simulink model "IOT_Charger"  (R2024b)
settings: Solver=ode23tb  StartTime=0.0  StopTime=1  RelTol=1e-3  EnableMultiTasking=on
PreLoadFcn:
  | % Data of Solar Panel
  | %5000[W]/130[W]
  | % Total power generated by solar panel reaches 5[KW].
  | % each solar panel generates power 130[kW].
  | V = [0    40 80 120 160 180 200 217 240 260 280];
  | I = 5000/130*[0.68 0.675 0.67 0.665 0.660 0.655 0.640 0.6 0.48 0.28 0];
  | 
  | %subplot(211);plot(V,I);xlabel('Voltage[V]');ylabel('Current[a]')
  | %subplot(212);plot(V.*I);title('Power[W]')
  | 
  | % Sample Time[s]
  | Ts =5e-6;
  | 
  | 
  | %MPPT + PV Control
  | % PI control pamameter of Voltage control(Outer loop)
  | Kp_V = 50e-3;
  | Ki_V = 10;
  | 
  | % PI Control pamameter of Current control(Inner loop)
  | Kp_I = 25e-3;
  | Ki_I = 10;
  | 
  | % Utility Interconnection Control
  | % PI Control pamameter of Voltage control(Outer loop)
  | Kp_V2 = 0.01;
  | Ki_V2 = 25;
  | 
  | % PI control pamameter of Current control(Inner loop)
  | Kp_I2 = 0.01;
  | Ki_I2 = 25;
  | 
  | 
  | % Difference of voltege using in MPPT
  | dV = 0.5;
  | 
  | % Battery Control
  | % PI Control pamameter of Voltage control(Outer loop)
  | Kp_VB = 0.4;
  | Ki_VB = 2;
  | 
  | % PI control pamameter of Current control(Inner loop)
  | Kp_IB = 0.1;
  | Ki_IB = 0.5;
undefined symbols (not defined in the file): Ion, Lithium, sigbuilder_block
libraries: spsBreakerLib x120, spsSeriesRLCBranchLib x72, spsBatteryLib x43, spsIdealSwitchLib x29, spsVoltageMeasurementLib x25, spsMosfetLib x19, slpidlib x17, spsSeriesRLCLoadLib x12, spsPWMGeneratorDCDCLib x11, spsCurrentMeasurementLib x10, spsDiodeLib x6, spsPWMGenerator2LevelLib x5
(part 6 of 6)

== matlab function IOT_Charger/MPPT and PV Controller/Swapping battery controller/MATLAB Function17 ==
  settings: updateMethod=DISCRETE
  data: SOC input; LoadOn output; ChargingOn output
function [LoadOn, ChargingOn] = chargeDischargeNode(SOC)
    % This function determines the charging and discharging states
    % based on the state of charge (SOC) of the battery.
    % Inputs:
    %   SOC - Current state of charge (0 to 100)
    % Outputs:
    %   LoadOn - Indicator if the load is on (1) or off (0)
    %   ChargingOn - Indicator if charging is active (1) or not (0)

    % Initialize persistent variables to retain state across function calls
    persistent LoadOnPersistent;
    persistent ChargingOnPersistent;

    if isempty(LoadOnPersistent)  % Initialize on first call
        LoadOnPersistent = 1;     % Load is initially on
        ChargingOnPersistent = 0;  % Charging is initially off
    end

    % Logic for charging and discharging based on SOC levels
    if SOC > 80
        LoadOnPersistent = 1;      % Turn load on if SOC is above 80%
        ChargingOnPersistent = 0;   % Turn charging off
    elseif SOC < 40
        LoadOnPersistent = 0;      % Turn load off if SOC is below 40%
        ChargingOnPersistent = 1;   % Start charging
    end

    % Assign output values from persistent variables
    LoadOn = LoadOnPersistent;
    ChargingOn = ChargingOnPersistent;
end

== matlab function IOT_Charger/MPPT and PV Controller/Swapping battery controller/MATLAB Function18 ==
  settings: updateMethod=DISCRETE
  data: SOC input; LoadOn output; ChargingOn output
function [LoadOn, ChargingOn] = chargeDischargeNode(SOC)
    % This function determines the charging and discharging states
    % based on the state of charge (SOC) of the battery.
    % Inputs:
    %   SOC - Current state of charge (0 to 100)
    % Outputs:
    %   LoadOn - Indicator if the load is on (1) or off (0)
    %   ChargingOn - Indicator if charging is active (1) or not (0)

    % Initialize persistent variables to retain state across function calls
    persistent LoadOnPersistent;
    persistent ChargingOnPersistent;

    if isempty(LoadOnPersistent)  % Initialize on first call
        LoadOnPersistent = 1;     % Load is initially on
        ChargingOnPersistent = 0;  % Charging is initially off
    end

    % Logic for charging and discharging based on SOC levels
    if SOC > 80
        LoadOnPersistent = 1;      % Turn load on if SOC is above 80%
        ChargingOnPersistent = 0;   % Turn charging off
    elseif SOC < 40
        LoadOnPersistent = 0;      % Turn load off if SOC is below 40%
        ChargingOnPersistent = 1;   % Start charging
    end

    % Assign output values from persistent variables
    LoadOn = LoadOnPersistent;
    ChargingOn = ChargingOnPersistent;
end

== matlab function IOT_Charger/MPPT and PV Controller/Swapping battery controller/MATLAB Function19 ==
  settings: updateMethod=DISCRETE
  data: SOC input; LoadOn output; ChargingOn output
function [LoadOn, ChargingOn] = chargeDischargeNode(SOC)
    % This function determines the charging and discharging states
    % based on the state of charge (SOC) of the battery.
    % Inputs:
    %   SOC - Current state of charge (0 to 100)
    % Outputs:
    %   LoadOn - Indicator if the load is on (1) or off (0)
    %   ChargingOn - Indicator if charging is active (1) or not (0)

    % Initialize persistent variables to retain state across function calls
    persistent LoadOnPersistent;
    persistent ChargingOnPersistent;

    if isempty(LoadOnPersistent)  % Initialize on first call
        LoadOnPersistent = 1;     % Load is initially on
        ChargingOnPersistent = 0;  % Charging is initially off
    end

    % Logic for charging and discharging based on SOC levels
    if SOC > 80
        LoadOnPersistent = 1;      % Turn load on if SOC is above 80%
        ChargingOnPersistent = 0;   % Turn charging off
    elseif SOC < 40
        LoadOnPersistent = 0;      % Turn load off if SOC is below 40%
        ChargingOnPersistent = 1;   % Start charging
    end

    % Assign output values from persistent variables
    LoadOn = LoadOnPersistent;
    ChargingOn = ChargingOnPersistent;
end

== matlab function IOT_Charger/MPPT and PV Controller/Swapping battery controller/MATLAB Function20 ==
  settings: updateMethod=DISCRETE
  data: SOC input; LoadOn output; ChargingOn output
function [LoadOn, ChargingOn] = chargeDischargeNode(SOC)
    % This function determines the charging and discharging states
    % based on the state of charge (SOC) of the battery.
    % Inputs:
    %   SOC - Current state of charge (0 to 100)
    % Outputs:
    %   LoadOn - Indicator if the load is on (1) or off (0)
    %   ChargingOn - Indicator if charging is active (1) or not (0)

    % Initialize persistent variables to retain state across function calls
    persistent LoadOnPersistent;
    persistent ChargingOnPersistent;

    if isempty(LoadOnPersistent)  % Initialize on first call
        LoadOnPersistent = 1;     % Load is initially on
        ChargingOnPersistent = 0;  % Charging is initially off
    end

    % Logic for charging and discharging based on SOC levels
    if SOC > 80
        LoadOnPersistent = 1;      % Turn load on if SOC is above 80%
        ChargingOnPersistent = 0;   % Turn charging off
    elseif SOC < 40
        LoadOnPersistent = 0;      % Turn load off if SOC is below 40%
        ChargingOnPersistent = 1;   % Start charging
    end

    % Assign output values from persistent variables
    LoadOn = LoadOnPersistent;
    ChargingOn = ChargingOnPersistent;
end

== matlab function IOT_Charger/MPPT and PV Controller/Swapping battery controller/MATLAB Function21 ==
  settings: updateMethod=DISCRETE
  data: SOC input; LoadOn output; ChargingOn output
function [LoadOn, ChargingOn] = chargeDischargeNode(SOC)
    % This function determines the charging and discharging states
    % based on the state of charge (SOC) of the battery.
    % Inputs:
    %   SOC - Current state of charge (0 to 100)
    % Outputs:
    %   LoadOn - Indicator if the load is on (1) or off (0)
    %   ChargingOn - Indicator if charging is active (1) or not (0)

    % Initialize persistent variables to retain state across function calls
    persistent LoadOnPersistent;
    persistent ChargingOnPersistent;

    if isempty(LoadOnPersistent)  % Initialize on first call
        LoadOnPersistent = 1;     % Load is initially on
        ChargingOnPersistent = 0;  % Charging is initially off
    end

    % Logic for charging and discharging based on SOC levels
    if SOC > 80
        LoadOnPersistent = 1;      % Turn load on if SOC is above 80%
        ChargingOnPersistent = 0;   % Turn charging off
    elseif SOC < 40
        LoadOnPersistent = 0;      % Turn load off if SOC is below 40%
        ChargingOnPersistent = 1;   % Start charging
    end

    % Assign output values from persistent variables
    LoadOn = LoadOnPersistent;
    ChargingOn = ChargingOnPersistent;
end

== matlab function IOT_Charger/MPPT and PV Controller/Swapping battery controller/MATLAB Function22 ==
  settings: updateMethod=DISCRETE
  data: SOC input; LoadOn output; ChargingOn output
function [LoadOn, ChargingOn] = chargeDischargeNode(SOC)
    % This function determines the charging and discharging states
    % based on the state of charge (SOC) of the battery.
    % Inputs:
    %   SOC - Current state of charge (0 to 100)
    % Outputs:
    %   LoadOn - Indicator if the load is on (1) or off (0)
    %   ChargingOn - Indicator if charging is active (1) or not (0)

    % Initialize persistent variables to retain state across function calls
    persistent LoadOnPersistent;
    persistent ChargingOnPersistent;

    if isempty(LoadOnPersistent)  % Initialize on first call
        LoadOnPersistent = 1;     % Load is initially on
        ChargingOnPersistent = 0;  % Charging is initially off
    end

    % Logic for charging and discharging based on SOC levels
    if SOC > 80
        LoadOnPersistent = 1;      % Turn load on if SOC is above 80%
        ChargingOnPersistent = 0;   % Turn charging off
    elseif SOC < 40
        LoadOnPersistent = 0;      % Turn load off if SOC is below 40%
        ChargingOnPersistent = 1;   % Start charging
    end

    % Assign output values from persistent variables
    LoadOn = LoadOnPersistent;
    ChargingOn = ChargingOnPersistent;
end

== matlab function IOT_Charger/MPPT and PV Controller/Swapping battery controller/MATLAB Function23 ==
  settings: updateMethod=DISCRETE
  data: SOC input; LoadOn output; ChargingOn output
function [LoadOn, ChargingOn] = chargeDischargeNode(SOC)
    % This function determines the charging and discharging states
    % based on the state of charge (SOC) of the battery.
    % Inputs:
    %   SOC - Current state of charge (0 to 100)
    % Outputs:
    %   LoadOn - Indicator if the load is on (1) or off (0)
    %   ChargingOn - Indicator if charging is active (1) or not (0)

    % Initialize persistent variables to retain state across function calls
    persistent LoadOnPersistent;
    persistent ChargingOnPersistent;

    if isempty(LoadOnPersistent)  % Initialize on first call
        LoadOnPersistent = 1;     % Load is initially on
        ChargingOnPersistent = 0;  % Charging is initially off
    end

    % Logic for charging and discharging based on SOC levels
    if SOC > 80
        LoadOnPersistent = 1;      % Turn load on if SOC is above 80%
        ChargingOnPersistent = 0;   % Turn charging off
    elseif SOC < 40
        LoadOnPersistent = 0;      % Turn load off if SOC is below 40%
        ChargingOnPersistent = 1;   % Start charging
    end

    % Assign output values from persistent variables
    LoadOn = LoadOnPersistent;
    ChargingOn = ChargingOnPersistent;
end

== matlab function IOT_Charger/MPPT and PV Controller/Swapping battery controller/MATLAB Function24 ==
  settings: updateMethod=DISCRETE
  data: SOC input; LoadOn output; ChargingOn output
function [LoadOn, ChargingOn] = chargeDischargeNode(SOC)
    % This function determines the charging and discharging states
    % based on the state of charge (SOC) of the battery.
    % Inputs:
    %   SOC - Current state of charge (0 to 100)
    % Outputs:
    %   LoadOn - Indicator if the load is on (1) or off (0)
    %   ChargingOn - Indicator if charging is active (1) or not (0)

    % Initialize persistent variables to retain state across function calls
    persistent LoadOnPersistent;
    persistent ChargingOnPersistent;

    if isempty(LoadOnPersistent)  % Initialize on first call
        LoadOnPersistent = 1;     % Load is initially on
        ChargingOnPersistent = 0;  % Charging is initially off
    end

    % Logic for charging and discharging based on SOC levels
    if SOC > 80
        LoadOnPersistent = 1;      % Turn load on if SOC is above 80%
        ChargingOnPersistent = 0;   % Turn charging off
    elseif SOC < 40
        LoadOnPersistent = 0;      % Turn load off if SOC is below 40%
        ChargingOnPersistent = 1;   % Start charging
    end

    % Assign output values from persistent variables
    LoadOn = LoadOnPersistent;
    ChargingOn = ChargingOnPersistent;
end

== matlab function IOT_Charger/MPPT and PV Controller/Swapping battery controller/MATLAB Function25 ==
  settings: updateMethod=DISCRETE
  data: SOC input; LoadOn output; ChargingOn output
function [LoadOn, ChargingOn] = chargeDischargeNode(SOC)
    % This function determines the charging and discharging states
    % based on the state of charge (SOC) of the battery.
    % Inputs:
    %   SOC - Current state of charge (0 to 100)
    % Outputs:
    %   LoadOn - Indicator if the load is on (1) or off (0)
    %   ChargingOn - Indicator if charging is active (1) or not (0)

    % Initialize persistent variables to retain state across function calls
    persistent LoadOnPersistent;
    persistent ChargingOnPersistent;

    if isempty(LoadOnPersistent)  % Initialize on first call
        LoadOnPersistent = 1;     % Load is initially on
        ChargingOnPersistent = 0;  % Charging is initially off
    end

    % Logic for charging and discharging based on SOC levels
    if SOC > 80
        LoadOnPersistent = 1;      % Turn load on if SOC is above 80%
        ChargingOnPersistent = 0;   % Turn charging off
    elseif SOC < 40
        LoadOnPersistent = 0;      % Turn load off if SOC is below 40%
        ChargingOnPersistent = 1;   % Start charging
    end

    % Assign output values from persistent variables
    LoadOn = LoadOnPersistent;
    ChargingOn = ChargingOnPersistent;
end

== matlab function IOT_Charger/MPPT and PV Controller/Swapping battery controller/MATLAB Function26 ==
  settings: updateMethod=DISCRETE
  data: SOC input; LoadOn output; ChargingOn output
function [LoadOn, ChargingOn] = chargeDischargeNode(SOC)
    % This function determines the charging and discharging states
    % based on the state of charge (SOC) of the battery.
    % Inputs:
    %   SOC - Current state of charge (0 to 100)
    % Outputs:
    %   LoadOn - Indicator if the load is on (1) or off (0)
    %   ChargingOn - Indicator if charging is active (1) or not (0)

    % Initialize persistent variables to retain state across function calls
    persistent LoadOnPersistent;
    persistent ChargingOnPersistent;

    if isempty(LoadOnPersistent)  % Initialize on first call
        LoadOnPersistent = 1;     % Load is initially on
        ChargingOnPersistent = 0;  % Charging is initially off
    end

    % Logic for charging and discharging based on SOC levels
    if SOC > 80
        LoadOnPersistent = 1;      % Turn load on if SOC is above 80%
        ChargingOnPersistent = 0;   % Turn charging off
    elseif SOC < 40
        LoadOnPersistent = 0;      % Turn load off if SOC is below 40%
        ChargingOnPersistent = 1;   % Start charging
    end

    % Assign output values from persistent variables
    LoadOn = LoadOnPersistent;
    ChargingOn = ChargingOnPersistent;
end

== matlab function IOT_Charger/MPPT and PV Controller/Swapping battery controller/MATLAB Function27 ==
  settings: updateMethod=DISCRETE
  data: SOC input; LoadOn output; ChargingOn output
function [LoadOn, ChargingOn] = chargeDischargeNode(SOC)
    % This function determines the charging and discharging states
    % based on the state of charge (SOC) of the battery.
    % Inputs:
    %   SOC - Current state of charge (0 to 100)
    % Outputs:
    %   LoadOn - Indicator if the load is on (1) or off (0)
    %   ChargingOn - Indicator if charging is active (1) or not (0)

    % Initialize persistent variables to retain state across function calls
    persistent LoadOnPersistent;
    persistent ChargingOnPersistent;

    if isempty(LoadOnPersistent)  % Initialize on first call
        LoadOnPersistent = 1;     % Load is initially on
        ChargingOnPersistent = 0;  % Charging is initially off
    end

    % Logic for charging and discharging based on SOC levels
    if SOC > 80
        LoadOnPersistent = 1;      % Turn load on if SOC is above 80%
        ChargingOnPersistent = 0;   % Turn charging off
    elseif SOC < 40
        LoadOnPersistent = 0;      % Turn load off if SOC is below 40%
        ChargingOnPersistent = 1;   % Start charging
    end

    % Assign output values from persistent variables
    LoadOn = LoadOnPersistent;
    ChargingOn = ChargingOnPersistent;
end

== matlab function IOT_Charger/MPPT and PV Controller/Swapping battery controller/MATLAB Function28 ==
  settings: updateMethod=DISCRETE
  data: SOC input; LoadOn output; ChargingOn output
function [LoadOn, ChargingOn] = chargeDischargeNode(SOC)
    % This function determines the charging and discharging states
    % based on the state of charge (SOC) of the battery.
    % Inputs:
    %   SOC - Current state of charge (0 to 100)
    % Outputs:
    %   LoadOn - Indicator if the load is on (1) or off (0)
    %   ChargingOn - Indicator if charging is active (1) or not (0)

    % Initialize persistent variables to retain state across function calls
    persistent LoadOnPersistent;
    persistent ChargingOnPersistent;

    if isempty(LoadOnPersistent)  % Initialize on first call
        LoadOnPersistent = 1;     % Load is initially on
        ChargingOnPersistent = 0;  % Charging is initially off
    end

    % Logic for charging and discharging based on SOC levels
    if SOC > 80
        LoadOnPersistent = 1;      % Turn load on if SOC is above 80%
        ChargingOnPersistent = 0;   % Turn charging off
    elseif SOC < 40
        LoadOnPersistent = 0;      % Turn load off if SOC is below 40%
        ChargingOnPersistent = 1;   % Start charging
    end

    % Assign output values from persistent variables
    LoadOn = LoadOnPersistent;
    ChargingOn = ChargingOnPersistent;
end

== matlab function IOT_Charger/MPPT and PV Controller/Swapping battery controller/MATLAB Function29 ==
  settings: updateMethod=DISCRETE
  data: SOC input; LoadOn output; ChargingOn output
function [LoadOn, ChargingOn] = chargeDischargeNode(SOC)
    % This function determines the charging and discharging states
    % based on the state of charge (SOC) of the battery.
    % Inputs:
    %   SOC - Current state of charge (0 to 100)
    % Outputs:
    %   LoadOn - Indicator if the load is on (1) or off (0)
    %   ChargingOn - Indicator if charging is active (1) or not (0)

    % Initialize persistent variables to retain state across function calls
    persistent LoadOnPersistent;
    persistent ChargingOnPersistent;

    if isempty(LoadOnPersistent)  % Initialize on first call
        LoadOnPersistent = 1;     % Load is initially on
        ChargingOnPersistent = 0;  % Charging is initially off
    end

    % Logic for charging and discharging based on SOC levels
    if SOC > 80
        LoadOnPersistent = 1;      % Turn load on if SOC is above 80%
        ChargingOnPersistent = 0;   % Turn charging off
    elseif SOC < 40
        LoadOnPersistent = 0;      % Turn load off if SOC is below 40%
        ChargingOnPersistent = 1;   % Start charging
    end

    % Assign output values from persistent variables
    LoadOn = LoadOnPersistent;
    ChargingOn = ChargingOnPersistent;
end

== matlab function IOT_Charger/Subsystem4/Subsystem/MATLAB Function ==
  data: u1 input; s1 output; u2 input; u3 input; s2 output; s3 output
function [s1, s2, s3] = fcn(u1, u2, u3)
    u1 = int32(u1);
    u2 = int32(u2);
    u3 = int32(u3);

    if (u1 > u2 || u1 > u3)
        s1 = 1;
    else
        s1 = 0;
    end

    if (u2 > u1 || u2 > u3)
        s2 = 1;
    else
        s2 = 0;
    end

    if (u3 > u1 || u3 > u2)
        s3 = 1;
    else
        s3 = 0;
    end
end

== matlab function IOT_Charger/Subsystem5/Subsystem/MATLAB Function ==
  data: u1 input; s1 output; u2 input; u3 input; s2 output; s3 output
function [s1, s2, s3] = fcn(u1, u2, u3)
    u1 = int32(u1);
    u2 = int32(u2);
    u3 = int32(u3);

    if (u1 > u2 || u1 > u3)
        s1 = 1;
    else
        s1 = 0;
    end

    if (u2 > u1 || u2 > u3)
        s2 = 1;
    else
        s2 = 0;
    end

    if (u3 > u1 || u3 > u2)
        s3 = 1;
    else
        s3 = 0;
    end
end

== matlab function IOT_Charger/Subsystem6/Subsystem/MATLAB Function ==
  data: u1 input; s1 output; u2 input; u3 input; s2 output; s3 output
function [s1, s2, s3] = fcn(u1, u2, u3)
    u1 = int32(u1);
    u2 = int32(u2);
    u3 = int32(u3);

    if (u1 > u2 || u1 > u3)
        s1 = 1;
    else
        s1 = 0;
    end

    if (u2 > u1 || u2 > u3)
        s2 = 1;
    else
        s2 = 0;
    end

    if (u3 > u1 || u3 > u2)
        s3 = 1;
    else
        s3 = 0;
    end
end

== matlab function IOT_Charger/Subsystem7/Subsystem/MATLAB Function ==
  data: u1 input; s1 output; u2 input; u3 input; s2 output; s3 output
function [s1, s2, s3] = fcn(u1, u2, u3)
    u1 = int32(u1);
    u2 = int32(u2);
    u3 = int32(u3);

    if (u1 > u2 || u1 > u3)
        s1 = 1;
    else
        s1 = 0;
    end

    if (u2 > u1 || u2 > u3)
        s2 = 1;
    else
        s2 = 0;
    end

    if (u3 > u1 || u3 > u2)
        s3 = 1;
    else
        s3 = 0;
    end
end

== matlab function IOT_Charger/Grid/Wall charger Connection Box/DC-AC // AC-DC Converter/Controller/MATLAB Function ==
  data: x input; a output; b output; ma input; shift input; c output
function [a,b,c] = ref_generation(x,ma,shift)

shift_k=shift*pi/180;
a=(ma*(sin((x)+shift_k)));
b=(ma*(sin((x)+shift_k-(2*pi/3))));
c=(ma*(sin((x)+shift_k+(2*pi/3))));

== stateflow chart IOT_Charger/MPPT and PV Controller/MMPT Controller/MPPT Controller ==
  settings: updateMethod=DISCRETE  sampleTime=5e-3
  state MPPT/
    (default) -> (junction 64)
    MPPT -> (junction 64)
    (junction 64) -> (junction 62) : {P_pv = I_pv*V_pv;}
    (junction 62) -> (junction 54) [order 2]
    (junction 62) -> (junction 61) [order 1] : [Last_P_pv >= P_pv]
        | {Vref = Vref - dV;}
    (junction 54) -> (junction 59) : [Last_P_pv < P_pv]
        | {Vref = Vref + dV;}
    (junction 59) -> (junction 61)
    (junction 61) -> (junction 52) : {Last_P_pv = P_pv;}
  (default) -> MPPT
  data: V_pv input; I_pv input; Last_P_pv local double; P_pv local double; Vref output double =200; dV parameter double
